simulink model "model"  (R2016b)
settings: Solver=ode14x  StartTime=0.0  StopTime=5  FixedStep=0.0001  RelTol=1e-3
values from neighbouring files (symbols this model uses):
  b = (Km*Kb/R)*((2*pi/60))^2    (= 2.64985465309e-07)    [params.m]
  J = 2.7*(10^(-7))    (= 2.7e-07)    [params.m]
  Kb = 0.00152/(2*pi/60)    (= 0.01451493081)    [params.m]
  Km = 0.0145    [params.m]
  L = 0.0002    [params.m]
  R = 8.71    [params.m]
settings Model: Creator=Mundt  LastModifiedBy=Mundt

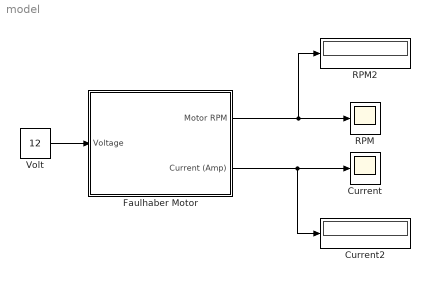
== system model ==
  Current : Scope
  Current2 : Display
  Faulhaber Motor : Subsystem
  RPM : Scope
  RPM2 : Display
  Volt : Constant  Value=12
  wires:
  Faulhaber Motor/1(Motor RPM) -> RPM2/1, RPM/1
  Volt/1 -> Faulhaber Motor/1(Voltage)
  Faulhaber Motor/2(Current (Amp)) -> Current2/1, Current/1

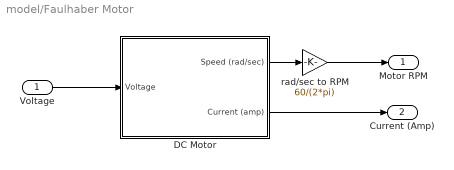
== system model/Faulhaber Motor ==
  Voltage : Inport
  DC Motor : Subsystem
  rad/sec to RPM : Gain  Gain=60/(2*pi)
  Motor RPM : Outport
  Current (Amp) : Outport  Port=2
  wires:
  DC Motor/2(Current (amp)) -> Current (Amp)/1
  DC Motor/1(Speed (rad/sec)) -> rad/sec to RPM/1
  rad/sec to RPM/1 -> Motor RPM/1
  Voltage/1 -> DC Motor/1(Voltage)

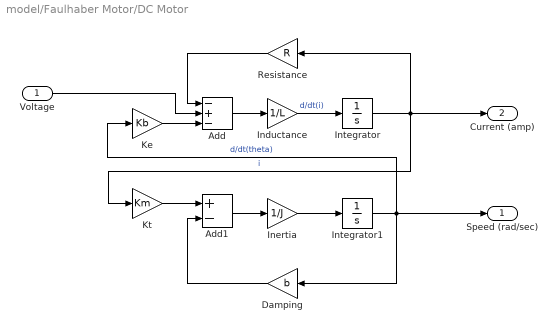
== system model/Faulhaber Motor/DC Motor ==
  Voltage : Inport
  Add : Sum  Inputs=-+-
  Add1 : Sum  Inputs=+-
  Damping : Gain  Gain=b
  Inductance : Gain  Gain=1/L
  Inertia : Gain  Gain=1/J
  Integrator : Integrator
  Integrator1 : Integrator
  Ke : Gain  Gain=Kb
  Kt : Gain  Gain=Km
  Resistance : Gain  Gain=R
  Speed (rad/sec) : Outport
  Current (amp) : Outport  Port=2
  wires:
  Resistance/1 -> Add/1
  Ke/1 -> Add/3
  Inertia/1 -> Integrator1/1
  Voltage/1 -> Add/2
  Damping/1 -> Add1/2
  Kt/1 -> Add1/1
  Add1/1 -> Inertia/1
  Inductance/1 -> Integrator/1  "d/dt(i)"
  Add/1 -> Inductance/1
  Integrator1/1 -> Speed (rad/sec)/1, Ke/1, Damping/1  "d/dt(theta)"
  Integrator/1 -> Current (amp)/1, Resistance/1, Kt/1  "i"
